simulink model "HiL"  (R2020b)
settings: Solver=VariableStepAuto  StartTime=0.0  StopTime=100  RelTol=1e-3
undefined symbols (not defined in the file): none, videoinput
libraries: dspvision x1, imaqlib x1, instrumentlib x1, slrealtimeiplib x1
settings Model: Creator=PranavUdhayakumar  LastModifiedBy=Capgemini Eng
settings DebuggingCC: UnconnectedInputMsg=none  UnconnectedOutputMsg=none  UnconnectedLineMsg=none
settings ModelReferenceCC: EnableRefExpFcnMdlSchedulingChecks=off

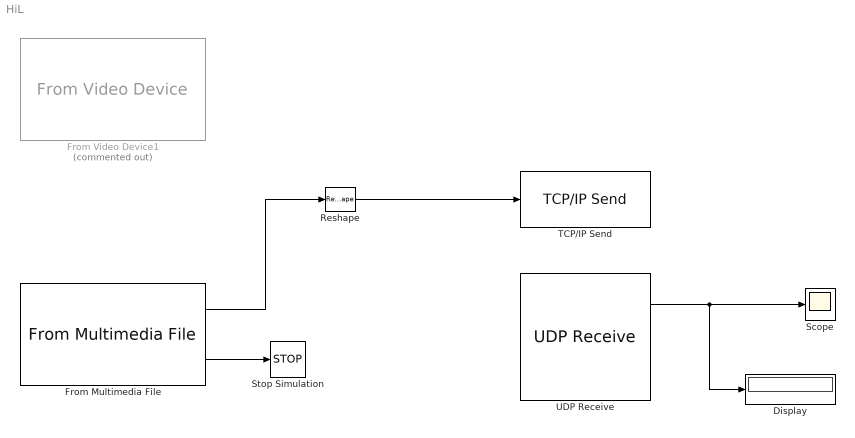
== system HiL ==
  Display : Display
  From Multimedia File : dspvision/From Multimedia File  inputFilename=C:\Program Files\MATLAB\R2020b\toolbox\vision\visiondata\visiontraffic.avi  readRange=[1 Inf]  loop=on  numPlays=1  outputStreams=Video only  videoDataType=uint8  audioDataType=int16  inheritSampleTime=off  userDefinedSampleTime=1/10  noAudioOutput=off  isIntensityVideo=off  fourcc=RGB  colorVideoFormat=One multidimensional signal  outputEOF=on  dataOrg=Column-major  audioFrameSize=1024  computeAudioFrameSize=off  outSamplingMode=Sample based
  From Video Device1 : imaqlib/From Video Device  Commented=on  DeviceMenu=winvideo 1 (USB Video Device)  Device=winvideo 1 (USB Video Device)  ObjConstructor=videoinput('winvideo', 1)  VideoFormatMenu=MJPG_640x360  VideoFormat=MJPG_640x360  VideoSource=input1  ROIPosition=[0 0 360 640]  EnableHWTrigger=off  TriggerConfiguration=none/none  SampleTime=0.01  OutputPortsMode=One multidimensional signal  DataType=uint8  CanDoHWTrigger=no  ReturnedColorSpace=rgb  BlockHandle=79.0001  ROIWidth=640  ROIHeight=360  ROIColumn=0  ROIRow=0  EngXMLPath=C:\Program Files\MATLAB\R2020b\toolbox\imaq\imaq\private  DevXMLPath=C:\ProgramData\MATLAB\SupportPackages\R2020b\toolbox\imaq\supportpackages\genericvideo\adaptor\win64  EngLibPath=C:\Program Files\MATLAB\R2020b\toolbox\imaq\imaqblks\imaqmex\win64  ColorSpace=rgb  BayerSensorAlignment=grbg  ImaqMode=on
  Reshape : Reshape
  Scope : Scope
  Stop Simulation : Stop
  TCP/IP Send : instrumentlib/TCP//IP Send  Priority=2  Host=192.168.0.2  Port=5005  EnableBlockingMode=on  Timeout=0.001  ByteOrder=LittleEndian  TransferDelay=off
  UDP Receive : slrealtimeiplib/UDP Receive  useHostTargetConn=off  ipAddress=192.168.0.1  localPort=5006  rcvWidth=1  rcvFmAny=on  fmAddress=10.10.10.10  rcvMulticast=off  multicastAddress={}  sampleTime=-1
      settings: SourceProductBaseCode=XP
  wires:
  Reshape/1 -> TCP/IP Send/1
  UDP Receive/1 -> Display/1, Scope/1
  From Multimedia File/1 -> Reshape/1
  From Multimedia File/2 -> Stop Simulation/1
